simulink model "Exercicio_8_Vinicius"  (R2018a)
settings: Solver=FixedStepAuto  StartTime=0.0  StopTime=40  FixedStep=Ts  RelTol=1e-3
undefined symbols (not defined in the file or in its folder): AA, Ax, B, BB, DD, H, KE, KF, KR, N, Nu, Ts, W
libraries: cstblocks x2, dspindex x2
settings Model: Creator=vinic  LastModifiedBy=vinic
settings SolverCC: AlgebraicLoopSolver=LineSearch

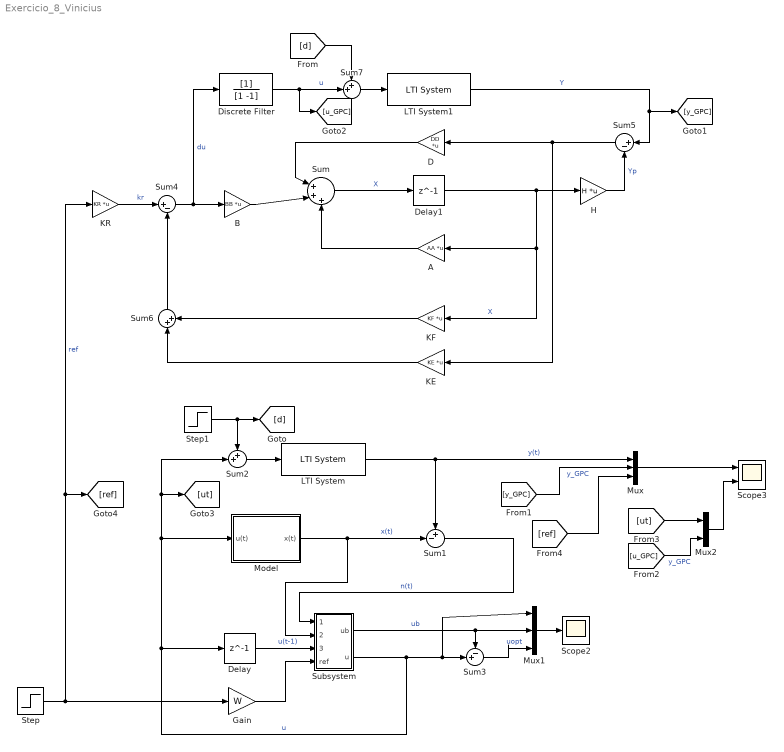
== system Exercicio_8_Vinicius ==
  A : Gain  Gain=AA  Multiplication=Matrix(K*u)
  B : Gain  Gain=BB  Multiplication=Matrix(K*u)
  D : Gain  Gain=DD  Multiplication=Matrix(K*u)
  Delay : Delay  DelayLength=1  SampleTime=Ts
  Delay1 : Delay  DelayLength=1  SampleTime=Ts
  Discrete Filter : DiscreteFilter  Denominator=[1 -1]  SampleTime=Ts
  Gain : Gain  Gain=W
  H : Gain  Gain=H  Multiplication=Matrix(K*u)
  KE : Gain  Gain=KE  Multiplication=Matrix(K*u)
  KF : Gain  Gain=KF  Multiplication=Matrix(K*u)
  KR : Gain  Gain=KR  Multiplication=Matrix(K*u)
  LTI System : cstblocks/LTI System  sys=Processo  IC=[]
  LTI System1 : cstblocks/LTI System  sys=Processo  IC=[]
  Model : Subsystem
  Mux : Mux  Inputs=3
  Mux1 : Mux  Inputs=3
  Mux2 : Mux  Inputs=2
  Scope2 : Scope
  Scope3 : Scope  NumInputPorts=2
  Step : Step  Time=0  SampleTime=Ts
  Step1 : Step  Time=10  After=0.1  SampleTime=Ts
  Subsystem : Subsystem
  Sum : Sum  Inputs=|+++
  Sum1 : Sum  Inputs=+-|
  Sum2 : Sum  Inputs=++|
  Sum3 : Sum  Inputs=-+|
  Sum4 : Sum  Inputs=|+-
  Sum5 : Sum  Inputs=|+-
  Sum6 : Sum  Inputs=|++
  Sum7 : Sum  Inputs=++|
  wires:
  LTI System/1 -> Mux/1, Sum1/1  "y(t)"
  Sum2/1 -> LTI System/1
  Step1/1 -> [d], Sum2/1
  Sum1/1 -> Subsystem/1(n(t))  "n(t)"
  Model/1(x(t)) -> Subsystem/2(x(t)), Sum1/2  "x(t)"
  Delay/1 -> Subsystem/3(u(t-1))  "u(t-1)"
  Subsystem/2(u) -> Mux1/1, Sum3/2, Model/1(u(t)), [ut], Sum2/2, Delay/1  "u"
  Gain/1 -> Subsystem/4(ref)
  Mux1/1 -> Scope2/1
  Subsystem/1(ub) -> Sum3/1, Mux1/2  "ub"
  Sum3/1 -> Mux1/3  "uopt"
  LTI System1/1 -> [y_GPC], Sum5/1  "Y"
  Sum4/1 -> Discrete Filter/1, B/1  "du"
  KR/1 -> Sum4/1  "kr"
  Sum6/1 -> Sum4/2
  Step/1 -> [ref], KR/1, Gain/1  "ref"
  D/1 -> Sum/1
  Delay1/1 -> KF/1, A/1, H/1  "X"
  A/1 -> Sum/3
  B/1 -> Sum/2
  KE/1 -> Sum6/1
  KF/1 -> Sum6/2
  H/1 -> Sum5/2  "Yp"
  Sum/1 -> Delay1/1  "X"
  Sum5/1 -> KE/1, D/1
  Discrete Filter/1 -> [u_GPC], Sum7/2  "u"
  Sum7/1 -> LTI System1/1
  [d] -> Sum7/1
  Mux/1 -> Scope3/1
  [y_GPC] -> Mux/2  "y_GPC"
  [u_GPC] -> Mux2/2  "y_GPC"
  [ut] -> Mux2/1
  Mux2/1 -> Scope3/2
  [ref] -> Mux/3

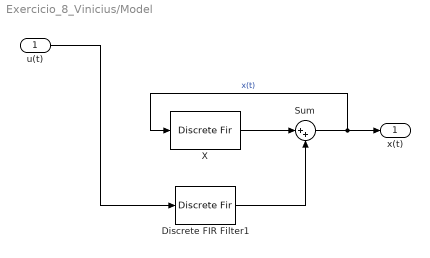
== system Exercicio_8_Vinicius/Model ==
  u(t) : Inport
  Discrete FIR Filter1 : DiscreteFir  Coefficients=[0 B]  SampleTime=Ts
  Sum : Sum  Inputs=|++
  X : DiscreteFir  Coefficients=[0 Ax]  SampleTime=Ts
  x(t) : Outport
  wires:
  Sum/1 -> x(t)/1, X/1  "x(t)"
  u(t)/1 -> Discrete FIR Filter1/1
  X/1 -> Sum/1
  Discrete FIR Filter1/1 -> Sum/2

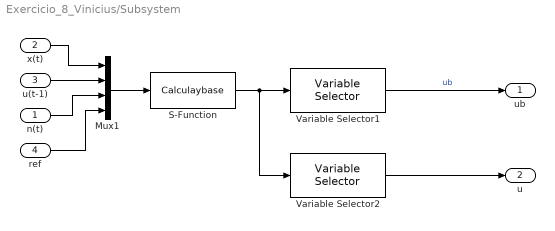
== system Exercicio_8_Vinicius/Subsystem ==
  n(t) : Inport
  x(t) : Inport  Port=2
  u(t-1) : Inport  Port=3
  ref : Inport  Port=4
  Mux1 : Mux
  S-Function : S-Function  FunctionName=Calculaybase  Parameters=Parametros  SFunctionDeploymentMode=off  EnableBusSupport=off
  Variable Selector1 : dspindex/Variable Selector  NumInputs=1  rowsOrCols=Columns  IdxMode=Fixed  Elements=1:1  ZerOneIdxMode=One-based  errmode=Clip Index  FillMode=on  FillValues=0
  Variable Selector2 : dspindex/Variable Selector  NumInputs=1  rowsOrCols=Columns  IdxMode=Fixed  Elements=N+Nu+1:N+Nu+1  ZerOneIdxMode=One-based  errmode=Clip Index  FillMode=on  FillValues=0
  ub : Outport
  u : Outport  Port=2
  wires:
  x(t)/1 -> Mux1/1
  u(t-1)/1 -> Mux1/2
  n(t)/1 -> Mux1/3
  Mux1/1 -> S-Function/1
  Variable Selector1/1 -> ub/1  "ub"
  S-Function/1 -> Variable Selector1/1, Variable Selector2/1
  Variable Selector2/1 -> u/1
  ref/1 -> Mux1/4
